simulink model "FOC_Sensorless"  (R2024a)
settings: Solver=FixedStepDiscrete  StartTime=0.0  StopTime=2  FixedStep=1e-7  RelTol=1e-3
libraries: simulink x3, spsDCVoltageSourceLib x1, spsGroundLib x1, spsPermanentMagnetSynchronousMachineLib x1, spsThreePhaseVIMeasurementLib x1, spsUniversalBridgeLib x1, spspowerguiLib x1
settings Model: Creator=lxcy  LastModifiedBy=lxcy

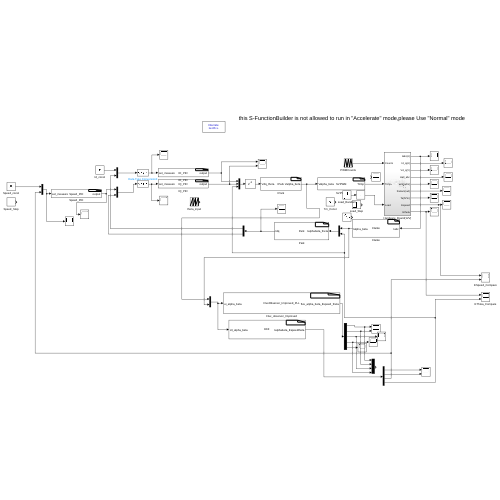
[thumbnail: Simulink's stored preview of the top-level diagram]
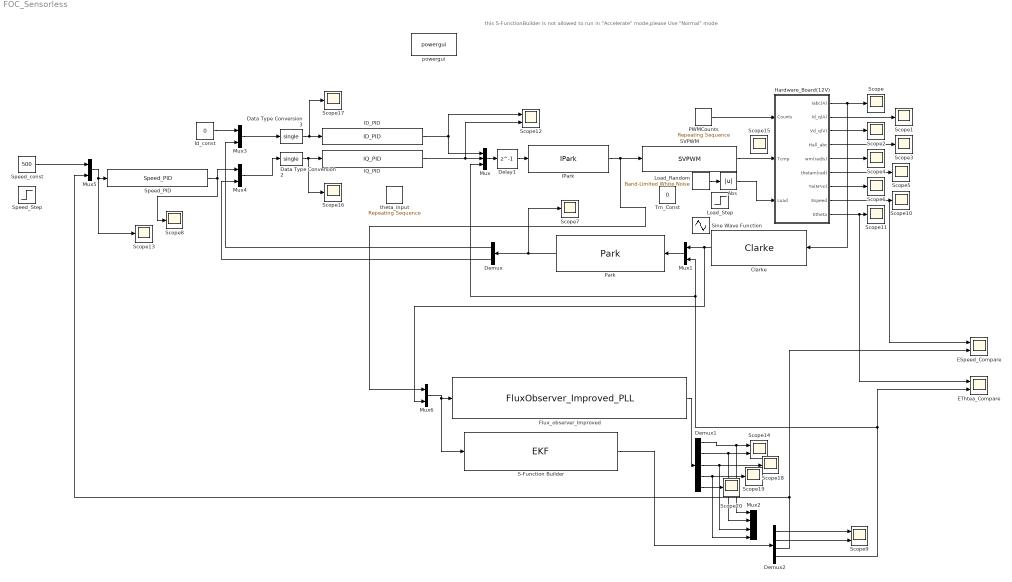
== system FOC_Sensorless ==
  note: this S-FunctionBuilder is not allowed to run in "Accelerate" mode,please Use "Normal" mode
  Abs : Abs  SaturateOnIntegerOverflow=off
  Clarke : S-Function  FunctionName=Clarke  SFunctionModules=Clarke_wrapper.c  SFunctionDeploymentMode=off  EnableBusSupport=off  mask(S-Function Builder){}
      mask help: Simulink:masks:SFunctionBuilder_MD
      mask init:
      | val = [[.9  0.75 0.75 1 1 .9 .9 1]',[1 1 0.75 0.75 .9 .9 1 .9]'];try , sys = get_param(gcb,'SfunBuilderFcnName');if isempty(sys), sys = get_param(gcb,'FunctionName'); end,catch, sys = get_param(gcb,'FunctionName'); end
      settings: CopyFcn=set_param(gcbh,'LinkStatus','none')  OpenFcn=sfunctionwizard(gcbh)
      mask Display:
      | plot(val(:,1),val(:,2))
      | disp(sys)
      | port_label('input',1,sprintf('%s', 'Iabc'),'interpreter','tex')
      | port_label('output',1,sprintf('%s', 'Ialpha\_beta'),'interpreter','tex')
  Data Type Conversion2 : DataTypeConversion  OutDataTypeStr=single  SaturateOnIntegerOverflow=off  RndMeth=Floor
  Data Type Conversion3 : DataTypeConversion  OutDataTypeStr=single  SaturateOnIntegerOverflow=off  RndMeth=Floor
  Delay1 : Delay  DelayLength=1  InitialCondition=0
  Demux : Demux  Outputs=2
  Demux1 : Demux  Outputs=5
  Demux2 : Demux
  ESpeed_Compare : Scope  NumInputPorts=2
  EThtea_Compare : Scope  NumInputPorts=2
  Flux_observer_Improved : S-Function  FunctionName=FluxObserver_Improved_PLL  SFunctionModules=FluxObserver_Improved_PLL_wrapper.c  SFunctionDeploymentMode=off  EnableBusSupport=off  mask(S-Function Builder){}
      mask help: Simulink:masks:SFunctionBuilder_MD
      mask init: same as FOC_Sensorless/Clarke
      settings: CopyFcn=set_param(gcbh,'LinkStatus','none')  OpenFcn=sfunctionwizard(gcbh)
      mask Display:
      | plot(val(:,1),val(:,2))
      | disp(sys)
      | port_label('input',1,sprintf('%s', 'ui\_alpha\_beta'),'interpreter','tex')
      | port_label('output',1,sprintf('%s', 'flux\_alpha\_beta\_Espeed\_theta'),'interpreter','tex')
  Hardware_Board(12V) : Subsystem
  ID_PID : S-Function  FunctionName=ID_PID  SFunctionModules=ID_PID_wrapper.c  SFunctionDeploymentMode=off  EnableBusSupport=off  mask(S-Function Builder){}
      mask help: Simulink:masks:SFunctionBuilder_MD
      mask init: same as FOC_Sensorless/Clarke
      settings: CopyFcn=set_param(gcbh,'LinkStatus','none')  OpenFcn=sfunctionwizard(gcbh)
      mask Display:
      | plot(val(:,1),val(:,2))
      | disp(sys)
      | port_label('input',1,sprintf('%s', 'set\_measure'),'interpreter','tex')
      | port_label('output',1,sprintf('%s', 'output'),'interpreter','tex')
  IPark : S-Function  FunctionName=IPark  SFunctionModules=IPark_wrapper.c  SFunctionDeploymentMode=off  EnableBusSupport=off  mask(S-Function Builder){}
      mask help: Simulink:masks:SFunctionBuilder_MD
      mask init: same as FOC_Sensorless/Clarke
      settings: CopyFcn=set_param(gcbh,'LinkStatus','none')  OpenFcn=sfunctionwizard(gcbh)
      mask Display:
      | plot(val(:,1),val(:,2))
      | disp(sys)
      | port_label('input',1,sprintf('%s', 'Vdq\_theta'),'interpreter','tex')
      | port_label('output',1,sprintf('%s', 'Valpha\_beta'),'interpreter','tex')
  IQ_PID : S-Function  FunctionName=IQ_PID  SFunctionModules=IQ_PID_wrapper.c  SFunctionDeploymentMode=off  EnableBusSupport=off  mask(S-Function Builder){}
      mask help: Simulink:masks:SFunctionBuilder_MD
      mask init: same as FOC_Sensorless/Clarke
      settings: CopyFcn=set_param(gcbh,'LinkStatus','none')  OpenFcn=sfunctionwizard(gcbh)
      mask Display:
      | plot(val(:,1),val(:,2))
      | disp(sys)
      | port_label('input',1,sprintf('%s', 'set\_measure'),'interpreter','tex')
      | port_label('output',1,sprintf('%s', 'output'),'interpreter','tex')
  Id_const : Constant  Value=0  OutDataTypeStr=single
  Load_Random : simulink/Sources/Band-Limited White Noise  Cov=[0.000000001]  Ts=1e-6  seed=[23341]
  Load_Step : Step  Time=0.7  Before=0.01  After=0.03  SampleTime=0
  Mux : Mux  Inputs=3
  Mux{1,3..6} (5 alike) : Mux  Inputs=2
  Mux2 : Mux
  PWMCounts : simulink/Sources/Repeating Sequence  rep_seq_t=[0 0.0001 0.0002]  rep_seq_y=[0 34000 0]
  Park : S-Function  FunctionName=Park  SFunctionModules=Park_wrapper.c  SFunctionDeploymentMode=off  EnableBusSupport=off  mask(S-Function Builder){}
      mask help: Simulink:masks:SFunctionBuilder_MD
      mask init: same as FOC_Sensorless/Clarke
      settings: CopyFcn=set_param(gcbh,'LinkStatus','none')  OpenFcn=sfunctionwizard(gcbh)
      mask Display:
      | plot(val(:,1),val(:,2))
      | disp(sys)
      | port_label('input',1,sprintf('%s', 'Ialphabeta\_theta'),'interpreter','tex')
      | port_label('output',1,sprintf('%s', 'Idq'),'interpreter','tex')
  S-Function Builder : S-Function  FunctionName=EKF  SFunctionModules=EKF_wrapper.c  SFunctionDeploymentMode=off  EnableBusSupport=off  mask(S-Function Builder){}
      mask help: Simulink:masks:SFunctionBuilder_MD
      mask init: same as FOC_Sensorless/Clarke
      settings: CopyFcn=set_param(gcbh,'LinkStatus','none')  OpenFcn=sfunctionwizard(gcbh)
      mask Display:
      | plot(val(:,1),val(:,2))
      | disp(sys)
      | port_label('input',1,sprintf('%s', 'UI\_alpha\_beta'),'interpreter','tex')
      | port_label('output',1,sprintf('%s', 'Ialphabeta\_Espeedtheta'),'interpreter','tex')
  SVPWM : S-Function  FunctionName=SVPWM  SFunctionModules=SVPWM_wrapper.c  SFunctionDeploymentMode=off  EnableBusSupport=off  mask(S-Function Builder){}
      mask help: Simulink:masks:SFunctionBuilder_MD
      mask init: same as FOC_Sensorless/Clarke
      settings: CopyFcn=set_param(gcbh,'LinkStatus','none')  OpenFcn=sfunctionwizard(gcbh)
      mask Display:
      | plot(val(:,1),val(:,2))
      | disp(sys)
      | port_label('input',1,sprintf('%s', 'Valpha\_beta'),'interpreter','tex')
      | port_label('output',1,sprintf('%s', 'Tcmp'),'interpreter','tex')
  Scope{,1..8,10..11,13,15..20} (18 alike) : Scope
  Scope12 : Scope  NumInputPorts=2
  Scope14 : Scope  NumInputPorts=2
  Scope9 : Scope  NumInputPorts=2
  Sine Wave Function : Sin  Amplitude=0.008  Bias=0.008  Frequency=50  SampleTime=0
  Speed_PID : S-Function  FunctionName=Speed_PID  SFunctionModules=Speed_PID_wrapper.c  SFunctionDeploymentMode=off  EnableBusSupport=off  mask(S-Function Builder){}
      mask help: Simulink:masks:SFunctionBuilder_MD
      mask init: same as FOC_Sensorless/Clarke
      settings: CopyFcn=set_param(gcbh,'LinkStatus','none')  OpenFcn=sfunctionwizard(gcbh)
      mask Display:
      | plot(val(:,1),val(:,2))
      | disp(sys)
      | port_label('input',1,sprintf('%s', 'set\_measure'),'interpreter','tex')
      | port_label('output',1,sprintf('%s', 'output'),'interpreter','tex')
  Speed_Step : Step  Time=0.3  Before=300  After=600  OutDataTypeStr=single  SampleTime=0
  Speed_const : Constant  Value=500  OutDataTypeStr=single
  Tm_Const : Constant  Value=0  OutDataTypeStr=double
  powergui : spspowerguiLib/powergui  Priority=1  SimulationMode=Discrete  SampleTime=1e-6  frequency=60  Iterations=50  frequencyindice=0  Pbase=100e6  ErrMax=1e-4  UnitsV=kV  UnitsW=MW  buscounter=0  FunctionMessages=off  echomessages=off  EnableUseOfTLC=off  CurrentSourceSwitches=off  DisableSnubberDevices=off  DisableRonSwitches=off  DisableVfSwitches=off  DisplayEquations=off  AutomaticDiscreteSolvers=off  SolverType=Tustin/Backward Euler (TBE)  Interpol=off  ExternalGateDelay=off  methode=off  Ts=100  x0status=blocks  SPID=on  SwTol=0  HookPort=off  NonlinearTolerance=1e-4  nMaxIteration=100  ContinueOnMaxIteration=off  RestoreLinks=warning  ResistiveCurrentMeasurement=off  Frange=[0:2:500]  Ylog=off  Xlog=on  ShowGrid=off  save=off  variable=ZData  structure=0  ZoomFFT=off  StartTime=0.0  cycles=1  DisplayStyle=1  fundamental=60  FreqAxis=off  MaxFrequency=1000  frequencyindicesteady=1  RmsSteady=1  display=off
  theta_input : simulink/Sources/Repeating Sequence  rep_seq_t=[0 0.1]  rep_seq_y=[0 2*pi]
  wires:
  PWMCounts/1 -> Hardware_Board(12V)/1(Counts)
  SVPWM/1 -> Hardware_Board(12V)/2(Tcmp)
  Hardware_Board(12V)/1(Iabc(A)) -> Clarke/1, Scope/1
  Hardware_Board(12V)/2(Id_q(A)) -> Scope1/1
  Hardware_Board(12V)/3(Vd_q(V)) -> Scope2/1
  Hardware_Board(12V)/4(Hall_abc) -> Scope3/1
  Hardware_Board(12V)/5(wm(rad/s)) -> Scope4/1
  Hardware_Board(12V)/6(thetam(rad)) -> Scope5/1
  Hardware_Board(12V)/7(Te(N*m)) -> Scope6/1
  Park/1 -> Scope7/1, Demux/1
  Mux1/1 -> Park/1
  Hardware_Board(12V)/8(Espeed) -> ESpeed_Compare/1, Scope10/1
  ID_PID/1 -> Mux/1, Scope12/1
  IQ_PID/1 -> Mux/2, Scope12/2
  Mux3/1 -> Data Type Conversion3/1
  Demux/1 -> Mux3/2
  Mux4/1 -> Data Type Conversion2/1
  Id_const/1 -> Mux3/1
  Demux/2 -> Mux4/2
  Data Type Conversion2/1 -> Scope16/1, IQ_PID/1
  Data Type Conversion3/1 -> Scope17/1, ID_PID/1
  Speed_PID/1 -> Mux4/1, Scope8/1
  Mux5/1 -> Scope13/1, Speed_PID/1
  Hardware_Board(12V)/9(Etheta) -> EThtea_Compare/1, Scope11/1
  Delay1/1 -> IPark/1
  Mux/1 -> Delay1/1
  Speed_const/1 -> Mux5/1
  Demux2/1 -> Scope9/1
  Demux2/2 -> Scope9/2
  Mux6/1 -> S-Function Builder/1, Flux_observer_Improved/1
  IPark/1 -> Mux6/1, SVPWM/1
  Clarke/1 -> Mux6/2, Mux1/1
  Load_Random/1 -> Abs/1
  Demux2/4 -> Mux/3, Mux1/2, EThtea_Compare/2
  Demux2/3 -> ESpeed_Compare/2, Mux5/2
  Flux_observer_Improved/1 -> Demux1/1
  Demux1/1 -> Mux2/1, Scope14/1
  Demux1/2 -> Mux2/2, Scope14/2
  Demux1/3 -> Mux2/3, Scope18/1
  Demux1/4 -> Mux2/4, Scope19/1
  Demux1/5 -> Scope20/1
  Abs/1 -> Hardware_Board(12V)/3(Load)
  S-Function Builder/1 -> Demux2/1

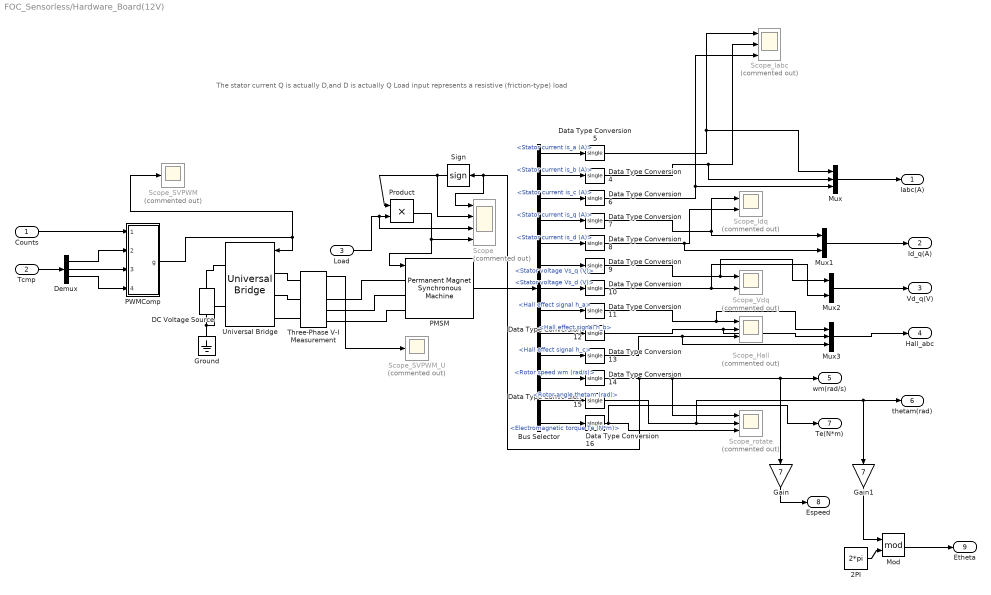
== system FOC_Sensorless/Hardware_Board(12V) ==
  note: The stator current Q is actually D,and D is actually Q
      | Load input represents a resistive (friction-type) load
  Counts : Inport
  Tcmp : Inport  Port=2
  Load : Inport  Port=3
  2PI : Constant  Value=2*pi  OutDataTypeStr=single
  Bus Selector : BusSelector  OutputSignals=Stator current is_a (A),Stator current is_b (A),Stator current is_c (A),Stator current is_q (A),Stator current is_d (A),Stator voltage Vs_q (V),Stator voltage Vs_d (V),Hall effect signal h_a,Hall effect signal h_b,Hall effect signal h_c,Rotor speed wm (rad/s),Rotor angle thetam (rad),Electromagnetic torque Te (N*m)
  DC Voltage Source : spsDCVoltageSourceLib/DC Voltage Source  Amplitude=12  Measurements=None
  Data Type Conversion{4..16} (13 alike) : DataTypeConversion  OutDataTypeStr=single  SaturateOnIntegerOverflow=off  RndMeth=Floor
  Demux : Demux  Outputs=3
  Gain : Gain  Gain=7
  Gain1 : Gain  Gain=7
  Ground : spsGroundLib/Ground  LConnTagsString=a
  Mod : Math  Operator=mod  OutputSignalType=real
  Mux : Mux  Inputs=3
  Mux1 : Mux  Inputs=2
  Mux2 : Mux  Inputs=2
  Mux3 : Mux  Inputs=3
  PMSM : spsPermanentMagnetSynchronousMachineLib/Permanent Magnet Synchronous Machine  NbPhases=3  FluxDistribution=Sinusoidal  RotorType=Round  MechanicalLoad=Torque Tm  PresetModel=No  ShowDetailedParameters=on  MeasurementBus=off  Resistance=5.5/2  Inductance=8.5e-3  dqInductances=[8.5e-3,8.5e-3]  La=2.0e-3/2  MachineConstant=Flux linkage established by magnets (V.s)  Flux=0.00386335  VoltageCst=4.9051  TorqueCst=0.040565  Flat=120  Mechanical=[1.764e-6,2e-5,7,0.0025]  PolePairs=4  InitialConditions=[0,0, 0,0]  InitialConditions5ph=[0 0 0 0 0 0]  RefAngle=Aligned with phase A axis (original Park)  IterativeDiscreteModel=Trapezoidal non iterative  TsBlock=-1  TsPowergui=0
  PWMComp : Subsystem
  Product : Product
  Scope : Scope  Commented=on  NumInputPorts=4
  Scope_Hall : Scope  Commented=on  NumInputPorts=3
  Scope_Iabc : Scope  Commented=on  NumInputPorts=3
  Scope_Idq : Scope  Commented=on  NumInputPorts=2
  Scope_SVPWM : Scope  Commented=on
  Scope_SVPWM_U : Scope  Commented=on
  Scope_Vdq : Scope  Commented=on  NumInputPorts=2
  Scope_rotate : Scope  Commented=on  NumInputPorts=3
  Sign : Signum
  Three-Phase V-I Measurement : spsThreePhaseVIMeasurementLib/Three-Phase V-I Measurement  VoltageMeasurement=phase-to-ground  SetLabelV=off  LabelV=Vabc  Vpu=off  VpuLL=off  CurrentMeasurement=yes  SetLabelI=off  LabelI=Iabc  Ipu=off  Pbase=100e6  Vbase=500e3  OutputType=Complex  PhasorSimulation=off  PSBequivalent=0
  Universal Bridge : spsUniversalBridgeLib/Universal Bridge  Arms=3  SnubberResistance=1e5  SnubberCapacitance=inf  Device=IGBT / Diodes  Ron=1e-3  Lon=0  ForwardVoltages="[  0  0  ]"  ForwardVoltage=0  GTOparameters=[ 10e-6 , 20e-6 ]  IGBTparameters=[ 1e-6 , 2e-6 ]  Measurements=None  Measurements_2=None  converterType=Rectifier
  Iabc(A) : Outport
  Id_q(A) : Outport  Port=2
  Vd_q(V) : Outport  Port=3
  Hall_abc : Outport  Port=4
  wm(rad/s) : Outport  Port=5
  thetam(rad) : Outport  Port=6
  Te(N*m) : Outport  Port=7
  Espeed : Outport  Port=8
  Etheta : Outport  Port=9
  wires:
  Demux/2 -> PWMComp/3(Tcmp2)
  Demux/1 -> PWMComp/2(Tcmp1)
  PMSM/1 -> Bus Selector/1
  Bus Selector/2 -> Data Type Conversion4/1  "<Stator current is_b (A)>"
  Bus Selector/8 -> Data Type Conversion11/1  "<Hall effect signal h_a>"
  Tcmp/1 -> Demux/1
  Data Type Conversion9/1 -> Mux2/1, Scope_Vdq/1
  Bus Selector/11 -> Data Type Conversion14/1  "<Rotor speed wm (rad/s)>"
  Demux/3 -> PWMComp/4(Tcmp3)
  Bus Selector/13 -> Data Type Conversion16/1  "<Electromagnetic torque Te (N*m)>"
  Mux3/1 -> Hall_abc/1
  Mux2/1 -> Vd_q(V)/1
  Mux1/1 -> Id_q(A)/1
  Mux/1 -> Iabc(A)/1
  Data Type Conversion16/1 -> Te(N*m)/1, Scope_rotate/3
  Data Type Conversion5/1 -> Mux/1, Scope_Iabc/1
  Bus Selector/7 -> Data Type Conversion10/1  "<Stator voltage Vs_d (V)>"
  Bus Selector/6 -> Data Type Conversion9/1  "<Stator voltage Vs_q (V)>"
  Data Type Conversion13/1 -> Mux3/3, Scope_Hall/3
  Data Type Conversion12/1 -> Mux3/2, Scope_Hall/2
  Bus Selector/1 -> Data Type Conversion5/1  "<Stator current is_a (A)>"
  PWMComp/1(g) -> Universal Bridge/1, Scope_SVPWM/1
  Data Type Conversion11/1 -> Mux3/1, Scope_Hall/1
  Data Type Conversion8/1 -> Mux1/2, Scope_Idq/2
  Bus Selector/4 -> Data Type Conversion7/1  "<Stator current is_q (A)>"
  Counts/1 -> PWMComp/1(Counts)
  Data Type Conversion4/1 -> Mux/2, Scope_Iabc/2
  Three-Phase V-I Measurement/1 -> Scope_SVPWM_U/1
  Bus Selector/12 -> Data Type Conversion15/1  "<Rotor angle thetam (rad)>"
  Data Type Conversion10/1 -> Mux2/2, Scope_Vdq/2
  Data Type Conversion15/1 -> Gain1/1, thetam(rad)/1, Scope_rotate/2
  Bus Selector/10 -> Data Type Conversion13/1  "<Hall effect signal h_c>"
  Bus Selector/9 -> Data Type Conversion12/1  "<Hall effect signal h_b>"
  Data Type Conversion6/1 -> Mux/3, Scope_Iabc/3
  Data Type Conversion7/1 -> Mux1/1, Scope_Idq/1
  Bus Selector/3 -> Data Type Conversion6/1  "<Stator current is_c (A)>"
  Bus Selector/5 -> Data Type Conversion8/1  "<Stator current is_d (A)>"
  Mod/1 -> Etheta/1
  2PI/1 -> Mod/2
  Gain1/1 -> Mod/1
  Gain/1 -> Espeed/1
  Sign/1 -> Product/1, Scope/2
  Load/1 -> Scope/3, Product/2
  Product/1 -> Scope/4, PMSM/1
  Data Type Conversion14/1 -> Sign/1, Scope/1, Gain/1, wm(rad/s)/1, Scope_rotate/1
  connections:
  PMSM/LConn2 -- Three-Phase V-I Measurement/RConn2
  Universal Bridge/LConn1 -- Three-Phase V-I Measurement/LConn1
  DC Voltage Source/RConn1 -- Universal Bridge/RConn1
  Universal Bridge/RConn2 -- DC Voltage Source/LConn1 -- Ground/LConn1
  Universal Bridge/LConn3 -- Three-Phase V-I Measurement/LConn3
  Universal Bridge/LConn2 -- Three-Phase V-I Measurement/LConn2
  Three-Phase V-I Measurement/RConn1 -- PMSM/LConn1
  Three-Phase V-I Measurement/RConn3 -- PMSM/LConn3

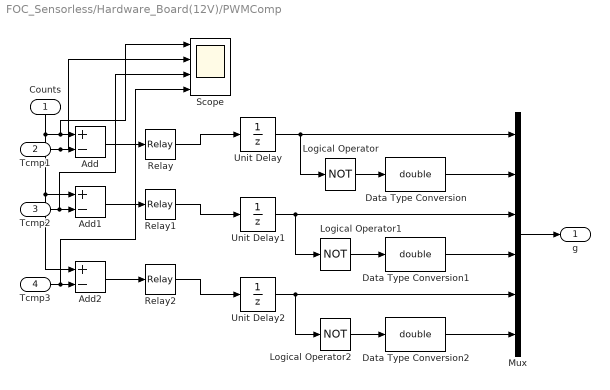
== system FOC_Sensorless/Hardware_Board(12V)/PWMComp ==
  Counts : Inport
  Tcmp1 : Inport  Port=2
  Tcmp2 : Inport  Port=3
  Tcmp3 : Inport  Port=4
  Add : Sum  Inputs=+-
  Add1 : Sum  Inputs=+-
  Add2 : Sum  Inputs=+-
  Data Type Conversion : DataTypeConversion  OutDataTypeStr=double  SaturateOnIntegerOverflow=off  RndMeth=Floor
  Data Type Conversion1 : DataTypeConversion  OutDataTypeStr=double  SaturateOnIntegerOverflow=off  RndMeth=Floor
  Data Type Conversion2 : DataTypeConversion  OutDataTypeStr=double  SaturateOnIntegerOverflow=off  RndMeth=Floor
  Logical Operator : Logic  Operator=NOT  AllPortsSameDT=off  OutDataTypeStr=boolean
  Logical Operator1 : Logic  Operator=NOT  AllPortsSameDT=off  OutDataTypeStr=boolean
  Logical Operator2 : Logic  Operator=NOT  AllPortsSameDT=off  OutDataTypeStr=boolean
  Mux : Mux  Inputs=6
  Relay : Relay  OffSwitchValue=-eps
  Relay1 : Relay  OffSwitchValue=-eps
  Relay2 : Relay  OffSwitchValue=-eps
  Scope : Scope  NumInputPorts=4
  Unit Delay : UnitDelay  SampleTime=-1  HasFrameUpgradeWarning=on
  Unit Delay1 : UnitDelay  SampleTime=-1  HasFrameUpgradeWarning=on
  Unit Delay2 : UnitDelay  SampleTime=-1  HasFrameUpgradeWarning=on
  g : Outport  VectorParamsAs1DForOutWhenUnconnected=off
  wires:
  Tcmp3/1 -> Scope/4, Add2/2
  Tcmp2/1 -> Scope/3, Add1/2
  Tcmp1/1 -> Scope/2, Add/2
  Relay2/1 -> Unit Delay2/1
  Relay1/1 -> Unit Delay1/1
  Relay/1 -> Unit Delay/1
  Unit Delay2/1 -> Mux/5, Logical Operator2/1
  Unit Delay1/1 -> Mux/3, Logical Operator1/1
  Unit Delay/1 -> Logical Operator/1, Mux/1
  Mux/1 -> g/1
  Data Type Conversion/1 -> Mux/2
  Data Type Conversion1/1 -> Mux/4
  Data Type Conversion2/1 -> Mux/6
  Logical Operator2/1 -> Data Type Conversion2/1
  Logical Operator1/1 -> Data Type Conversion1/1
  Logical Operator/1 -> Data Type Conversion/1
  Add1/1 -> Relay1/1
  Add2/1 -> Relay2/1
  Add/1 -> Relay/1
  Counts/1 -> Scope/1, Add/1, Add2/1, Add1/1
